simulink model "SecRwLtStLtwdRtwdTrgtPosSelc"  (R2018b)
settings: Solver=FixedStepDiscrete  StartTime=0.0  StopTime=10.0  FixedStep=0.01  RelTol=1e-3
undefined symbols (not defined in the file or in its folder): KeSMSw6sAcsEntrySecRwLtStLtwdRtwdPos_Val, KeSMSw6sAcsEntrySecRwLtStLtwdRtwdPosMax_Val, KeSMSw6sAcsEntrySecRwLtStLtwdRtwdPosMin_Val, KeSMSw6sAcsExtSecRwLtStLtwdRtwdPos_Val, KeSMSw6sAcsExtSecRwLtStLtwdRtwdPosMax_Val, KeSMSw6sAcsExtSecRwLtStLtwdRtwdPosMin_Val, KeSMSw6sFamilyMdSecRwLtStLtwdRtwdPos_Val, KeSMSw6sFamilyMdSecRwLtStLtwdRtwdPosMax_Val, KeSMSw6sFamilyMdSecRwLtStLtwdRtwdPosMin_Val, KeSMSw6sFamilyRMdSecRwLtStLtwdRtwdPos_Val, KeSMSw6sFamilyRMdSecRwLtStLtwdRtwdPosMax_Val, KeSMSw6sFamilyRMdSecRwLtStLtwdRtwdPosMin_Val, KeSMSw6sIntimacyMdSecRwLtStLtwdRtwdPos_Val, KeSMSw6sIntimacyMdSecRwLtStLtwdRtwdPosMax_Val, KeSMSw6sIntimacyMdSecRwLtStLtwdRtwdPosMin_Val, KeSMSw6sIntimacyRMdSecRwLtStLtwdRtwdPos_Val, KeSMSw6sIntimacyRMdSecRwLtStLtwdRtwdPosMax_Val, KeSMSw6sIntimacyRMdSecRwLtStLtwdRtwdPosMin_Val, KeSMSw6sVIPSecRwLtStLtwdRtwdPos_Val, KeSMSw6sVIPSecRwLtStLtwdRtwdPosMax_Val, KeSMSw6sVIPSecRwLtStLtwdRtwdPosMin_Val, KeSMSwAcsEntrySecRwLtStLtwdRtwdPos_Val, KeSMSwAcsEntrySecRwLtStLtwdRtwdPosMax_Val, KeSMSwAcsEntrySecRwLtStLtwdRtwdPosMin_Val, KeSMSwAcsExtSecRwLtStLtwdRtwdPos_Val, KeSMSwAcsExtSecRwLtStLtwdRtwdPosMax_Val, KeSMSwAcsExtSecRwLtStLtwdRtwdPosMin_Val, KeSMSwFamilyMdSecRwLtStLtwdRtwdPos_Val, KeSMSwFamilyMdSecRwLtStLtwdRtwdPosMax_Val, KeSMSwFamilyMdSecRwLtStLtwdRtwdPosMin_Val, KeSMSwFamilyRMdSecRwLtStLtwdRtwdPos_Val, KeSMSwFamilyRMdSecRwLtStLtwdRtwdPosMax_Val, KeSMSwFamilyRMdSecRwLtStLtwdRtwdPosMin_Val, KeSMSwIntimacyMdSecRwLtStLtwdRtwdPos_Val, KeSMSwIntimacyMdSecRwLtStLtwdRtwdPosMax_Val, KeSMSwIntimacyMdSecRwLtStLtwdRtwdPosMin_Val, KeSMSwIntimacyRMdSecRwLtStLtwdRtwdPos_Val, KeSMSwIntimacyRMdSecRwLtStLtwdRtwdPosMax_Val, KeSMSwIntimacyRMdSecRwLtStLtwdRtwdPosMin_Val, KeSMSwVIPSecRwLtStLtwdRtwdPos_Val, KeSMSwVIPSecRwLtStLtwdRtwdPosMax_Val, KeSMSwVIPSecRwLtStLtwdRtwdPosMin_Val
libraries: TrgtPosSelcLib x8
settings Model: Creator=sn2xws  LastModifiedBy=sn2xws
settings DataIOCC: SaveFormat=StructureWithTime
settings OptimizationCC: DefaultParameterBehavior=Inlined  EnhancedBackFolding=on  PassReuseOutputArgsAs=Individual arguments  ZeroExternalMemoryAtStartup=off  ZeroInternalMemoryAtStartup=off  OptimizeBlockOrder=speed  DifferentSizesBufferReuse=on  OptimizationCustomize=off
settings DebuggingCC: ParameterTunabilityLossMsg=error
settings ModelReferenceCC: ModelReferenceNumInstancesAllowed=Single
settings SFSimCC: MATLABDynamicMemAlloc=off
settings RTWCC: SystemTargetFile=autosar.tlc  GenCodeOnly=on  TemplateMakefile=ert_default_tmf  Description=AUTOSAR  GenerateReport=on  IncludeHyperlinkInReport=on  LaunchReport=on  GenerateTraceInfo=on  GenerateTraceReport=on  GenerateTraceReportSl=on  GenerateTraceReportSf=on  GenerateTraceReportEml=on
settings CodeAppCC: ForceParamTrailComments=on  IgnoreCustomStorageClasses=off  OperatorAnnotations=on  SimulinkDataObjDesc=on  SFDataObjDesc=on  InsertBlockDesc=on
settings STFCustomTargetCC: TargetLangStandard=C99 (ISO)  MultiwordLength=256  ParMdlRefBuildCompliant=on  CompOptLevelCompliant=on  IncludeMdlTerminateFcn=off  CombineOutputUpdateFcns=on  SuppressErrorStatus=on  ERTCustomFileBanners=on  SupportNonFinite=off  SupportComplex=off  SupportContinuousTime=off  SupportNonInlinedSFcns=off  RemoveResetFunc=on  MATLABClassNameForMDSCustomization=Simulink.SoftwareTarget.ERTCustomization  AutosarCompliant=on  UseToolchainInfoCompliant=on  LookupTableObjectStructAxisOrder=2,1,3,4,...  LUTObjectStructOrderEvenSpacing=Size,Table,Breakpoints  SystemTargetFile=autosar.tlc
settings ERTTargetCC: TargetLangStandard=C99 (ISO)  ConcurrentExecutionCompliant=off  IncludeMdlTerminateFcn=off  SuppressErrorStatus=on  SupportNonFinite=off  SupportComplex=off  ModelStepFunctionPrototypeControlCompliant=off  CPPClassGenCompliant=off  AutosarCompliant=on  LookupTableObjectStructAxisOrder=2,1,3,4,...  LUTObjectStructOrderEvenSpacing=Size,Table,Breakpoints  InlinedParameterPlacement=NonHierarchical  ERTCustomFileTemplate=example_file_process.tlc  ERTFilePackagingFormat=Compact

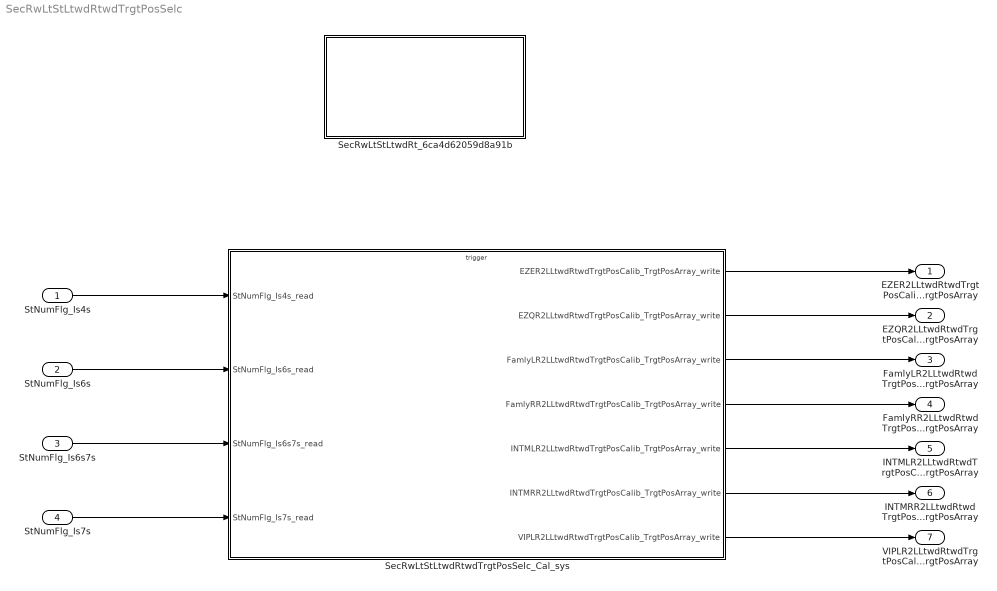
== system SecRwLtStLtwdRtwdTrgtPosSelc ==
  StNumFlg_Is4s : Inport  OutDataTypeStr=boolean  PortDimensions=1
  StNumFlg_Is6s : Inport  Port=2  OutDataTypeStr=boolean  PortDimensions=1
  StNumFlg_Is6s7s : Inport  Port=3  OutDataTypeStr=boolean  PortDimensions=1
  StNumFlg_Is7s : Inport  Port=4  OutDataTypeStr=boolean  PortDimensions=1
  SecRwLtStLtwdRt_6ca4d62059d8a91b : Subsystem
  SecRwLtStLtwdRtwdTrgtPosSelc_Cal_sys : Subsystem
  EZER2LLtwdRtwdTrgtPosCalib_TrgtPosArray : Outport  Description=|  OutDataTypeStr=uint16  PortDimensions=3
      | 0:Pos
      | 1:Max
      | 2:Min
  EZQR2LLtwdRtwdTrgtPosCalib_TrgtPosArray : Outport  Description=|  Port=2  OutDataTypeStr=uint16  PortDimensions=3
      | 0:Pos
      | 1:Max
      | 2:Min
  FamlyLR2LLtwdRtwdTrgtPosCalib_TrgtPosArray : Outport  Description=|  Port=3  OutDataTypeStr=uint16  PortDimensions=3
      | 0:Pos
      | 1:Max
      | 2:Min
  FamlyRR2LLtwdRtwdTrgtPosCalib_TrgtPosArray : Outport  Description=|  Port=4  OutDataTypeStr=uint16  PortDimensions=3
      | 0:Pos
      | 1:Max
      | 2:Min
  INTMLR2LLtwdRtwdTrgtPosCalib_TrgtPosArray : Outport  Description=|  Port=5  OutDataTypeStr=uint16  PortDimensions=3
      | 0:Pos
      | 1:Max
      | 2:Min
  INTMRR2LLtwdRtwdTrgtPosCalib_TrgtPosArray : Outport  Description=|  Port=6  OutDataTypeStr=uint16  PortDimensions=3
      | 0:Pos
      | 1:Max
      | 2:Min
  VIPLR2LLtwdRtwdTrgtPosCalib_TrgtPosArray : Outport  Description=|  Port=7  OutDataTypeStr=uint16  PortDimensions=3
      | 0:Pos
      | 1:Max
      | 2:Min
  wires:
  StNumFlg_Is4s/1 -> SecRwLtStLtwdRtwdTrgtPosSelc_Cal_sys/1(StNumFlg_Is4s_read)
  StNumFlg_Is6s/1 -> SecRwLtStLtwdRtwdTrgtPosSelc_Cal_sys/2(StNumFlg_Is6s_read)
  StNumFlg_Is6s7s/1 -> SecRwLtStLtwdRtwdTrgtPosSelc_Cal_sys/3(StNumFlg_Is6s7s_read)
  StNumFlg_Is7s/1 -> SecRwLtStLtwdRtwdTrgtPosSelc_Cal_sys/4(StNumFlg_Is7s_read)
  SecRwLtStLtwdRtwdTrgtPosSelc_Cal_sys/1(EZER2LLtwdRtwdTrgtPosCalib_TrgtPosArray_write) -> EZER2LLtwdRtwdTrgtPosCalib_TrgtPosArray/1
  SecRwLtStLtwdRtwdTrgtPosSelc_Cal_sys/2(EZQR2LLtwdRtwdTrgtPosCalib_TrgtPosArray_write) -> EZQR2LLtwdRtwdTrgtPosCalib_TrgtPosArray/1
  SecRwLtStLtwdRtwdTrgtPosSelc_Cal_sys/3(FamlyLR2LLtwdRtwdTrgtPosCalib_TrgtPosArray_write) -> FamlyLR2LLtwdRtwdTrgtPosCalib_TrgtPosArray/1
  SecRwLtStLtwdRtwdTrgtPosSelc_Cal_sys/4(FamlyRR2LLtwdRtwdTrgtPosCalib_TrgtPosArray_write) -> FamlyRR2LLtwdRtwdTrgtPosCalib_TrgtPosArray/1
  SecRwLtStLtwdRtwdTrgtPosSelc_Cal_sys/5(INTMLR2LLtwdRtwdTrgtPosCalib_TrgtPosArray_write) -> INTMLR2LLtwdRtwdTrgtPosCalib_TrgtPosArray/1
  SecRwLtStLtwdRtwdTrgtPosSelc_Cal_sys/6(INTMRR2LLtwdRtwdTrgtPosCalib_TrgtPosArray_write) -> INTMRR2LLtwdRtwdTrgtPosCalib_TrgtPosArray/1
  SecRwLtStLtwdRtwdTrgtPosSelc_Cal_sys/7(VIPLR2LLtwdRtwdTrgtPosCalib_TrgtPosArray_write) -> VIPLR2LLtwdRtwdTrgtPosCalib_TrgtPosArray/1

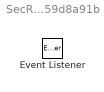
== system SecRwLtStLtwdRtwdTrgtPosSelc/SecRwLtStLtwdRt_6ca4d62059d8a91b ==
  Event Listener : EventListener  EventName=reset

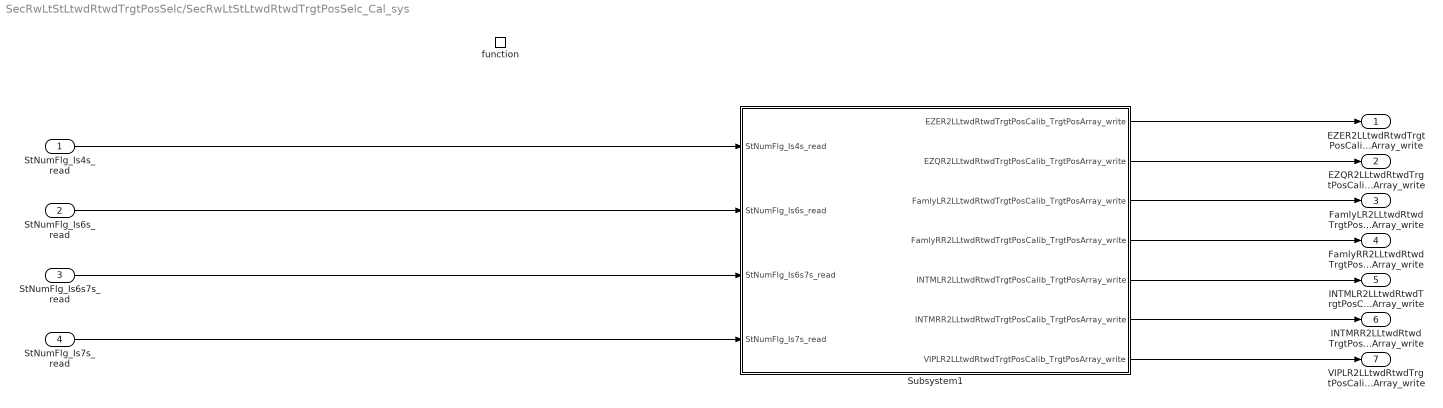
== system SecRwLtStLtwdRtwdTrgtPosSelc/SecRwLtStLtwdRtwdTrgtPosSelc_Cal_sys ==
  StNumFlg_Is4s_read : Inport
  StNumFlg_Is6s_read : Inport  Port=2
  StNumFlg_Is6s7s_read : Inport  Port=3
  StNumFlg_Is7s_read : Inport  Port=4
  function : TriggerPort  TriggerType=function-call  IsSimulinkFunction=on  FunctionName=SecRwLtStLtwdRtwdTrgtPosSelc_Cal  VariantControl=(inherit)
  Subsystem1 : Subsystem
  EZER2LLtwdRtwdTrgtPosCalib_TrgtPosArray_write : Outport
      settings: EnsureOutportIsVirtual=on
  EZQR2LLtwdRtwdTrgtPosCalib_TrgtPosArray_write : Outport  Port=2
      settings: EnsureOutportIsVirtual=on
  FamlyLR2LLtwdRtwdTrgtPosCalib_TrgtPosArray_write : Outport  Port=3
      settings: EnsureOutportIsVirtual=on
  FamlyRR2LLtwdRtwdTrgtPosCalib_TrgtPosArray_write : Outport  Port=4
      settings: EnsureOutportIsVirtual=on
  INTMLR2LLtwdRtwdTrgtPosCalib_TrgtPosArray_write : Outport  Port=5
      settings: EnsureOutportIsVirtual=on
  INTMRR2LLtwdRtwdTrgtPosCalib_TrgtPosArray_write : Outport  Port=6
      settings: EnsureOutportIsVirtual=on
  VIPLR2LLtwdRtwdTrgtPosCalib_TrgtPosArray_write : Outport  Port=7
      settings: EnsureOutportIsVirtual=on
  wires:
  Subsystem1/1(EZER2LLtwdRtwdTrgtPosCalib_TrgtPosArray_write) -> EZER2LLtwdRtwdTrgtPosCalib_TrgtPosArray_write/1
  Subsystem1/2(EZQR2LLtwdRtwdTrgtPosCalib_TrgtPosArray_write) -> EZQR2LLtwdRtwdTrgtPosCalib_TrgtPosArray_write/1
  Subsystem1/3(FamlyLR2LLtwdRtwdTrgtPosCalib_TrgtPosArray_write) -> FamlyLR2LLtwdRtwdTrgtPosCalib_TrgtPosArray_write/1
  Subsystem1/4(FamlyRR2LLtwdRtwdTrgtPosCalib_TrgtPosArray_write) -> FamlyRR2LLtwdRtwdTrgtPosCalib_TrgtPosArray_write/1
  Subsystem1/5(INTMLR2LLtwdRtwdTrgtPosCalib_TrgtPosArray_write) -> INTMLR2LLtwdRtwdTrgtPosCalib_TrgtPosArray_write/1
  Subsystem1/6(INTMRR2LLtwdRtwdTrgtPosCalib_TrgtPosArray_write) -> INTMRR2LLtwdRtwdTrgtPosCalib_TrgtPosArray_write/1
  Subsystem1/7(VIPLR2LLtwdRtwdTrgtPosCalib_TrgtPosArray_write) -> VIPLR2LLtwdRtwdTrgtPosCalib_TrgtPosArray_write/1
  StNumFlg_Is4s_read/1 -> Subsystem1/1(StNumFlg_Is4s_read)
  StNumFlg_Is6s_read/1 -> Subsystem1/2(StNumFlg_Is6s_read)
  StNumFlg_Is6s7s_read/1 -> Subsystem1/3(StNumFlg_Is6s7s_read)
  StNumFlg_Is7s_read/1 -> Subsystem1/4(StNumFlg_Is7s_read)

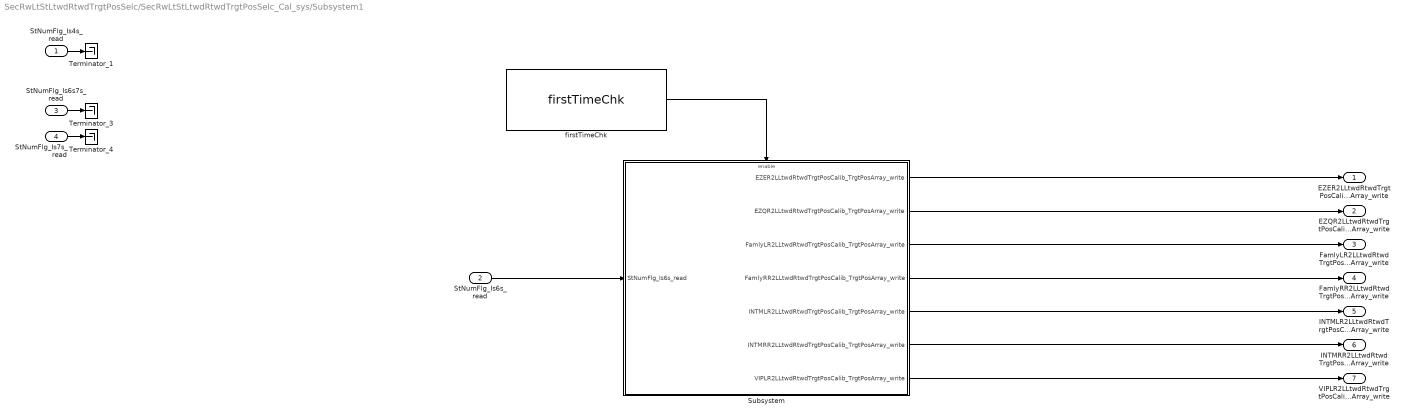
== system SecRwLtStLtwdRtwdTrgtPosSelc/SecRwLtStLtwdRtwdTrgtPosSelc_Cal_sys/Subsystem1 ==
  StNumFlg_Is4s_read : Inport
  StNumFlg_Is6s_read : Inport  Port=2
  StNumFlg_Is6s7s_read : Inport  Port=3
  StNumFlg_Is7s_read : Inport  Port=4
  Subsystem : Subsystem
  Terminator_1 : Terminator
  Terminator_3 : Terminator
  Terminator_4 : Terminator
  firstTimeChk : TrgtPosSelcLib/firstTimeChk  SystemSampleTime=-1
  EZER2LLtwdRtwdTrgtPosCalib_TrgtPosArray_write : Outport
      settings: EnsureOutportIsVirtual=on
  EZQR2LLtwdRtwdTrgtPosCalib_TrgtPosArray_write : Outport  Port=2
      settings: EnsureOutportIsVirtual=on
  FamlyLR2LLtwdRtwdTrgtPosCalib_TrgtPosArray_write : Outport  Port=3
      settings: EnsureOutportIsVirtual=on
  FamlyRR2LLtwdRtwdTrgtPosCalib_TrgtPosArray_write : Outport  Port=4
      settings: EnsureOutportIsVirtual=on
  INTMLR2LLtwdRtwdTrgtPosCalib_TrgtPosArray_write : Outport  Port=5
      settings: EnsureOutportIsVirtual=on
  INTMRR2LLtwdRtwdTrgtPosCalib_TrgtPosArray_write : Outport  Port=6
      settings: EnsureOutportIsVirtual=on
  VIPLR2LLtwdRtwdTrgtPosCalib_TrgtPosArray_write : Outport  Port=7
      settings: EnsureOutportIsVirtual=on
  wires:
  StNumFlg_Is4s_read/1 -> Terminator_1/1
  StNumFlg_Is6s7s_read/1 -> Terminator_3/1
  Subsystem/6(INTMRR2LLtwdRtwdTrgtPosCalib_TrgtPosArray_write) -> INTMRR2LLtwdRtwdTrgtPosCalib_TrgtPosArray_write/1
  Subsystem/3(FamlyLR2LLtwdRtwdTrgtPosCalib_TrgtPosArray_write) -> FamlyLR2LLtwdRtwdTrgtPosCalib_TrgtPosArray_write/1
  Subsystem/1(EZER2LLtwdRtwdTrgtPosCalib_TrgtPosArray_write) -> EZER2LLtwdRtwdTrgtPosCalib_TrgtPosArray_write/1
  Subsystem/2(EZQR2LLtwdRtwdTrgtPosCalib_TrgtPosArray_write) -> EZQR2LLtwdRtwdTrgtPosCalib_TrgtPosArray_write/1
  Subsystem/5(INTMLR2LLtwdRtwdTrgtPosCalib_TrgtPosArray_write) -> INTMLR2LLtwdRtwdTrgtPosCalib_TrgtPosArray_write/1
  Subsystem/4(FamlyRR2LLtwdRtwdTrgtPosCalib_TrgtPosArray_write) -> FamlyRR2LLtwdRtwdTrgtPosCalib_TrgtPosArray_write/1
  Subsystem/7(VIPLR2LLtwdRtwdTrgtPosCalib_TrgtPosArray_write) -> VIPLR2LLtwdRtwdTrgtPosCalib_TrgtPosArray_write/1
  StNumFlg_Is7s_read/1 -> Terminator_4/1
  StNumFlg_Is6s_read/1 -> Subsystem/1(StNumFlg_Is6s_read)
  firstTimeChk/1 -> Subsystem/Enable

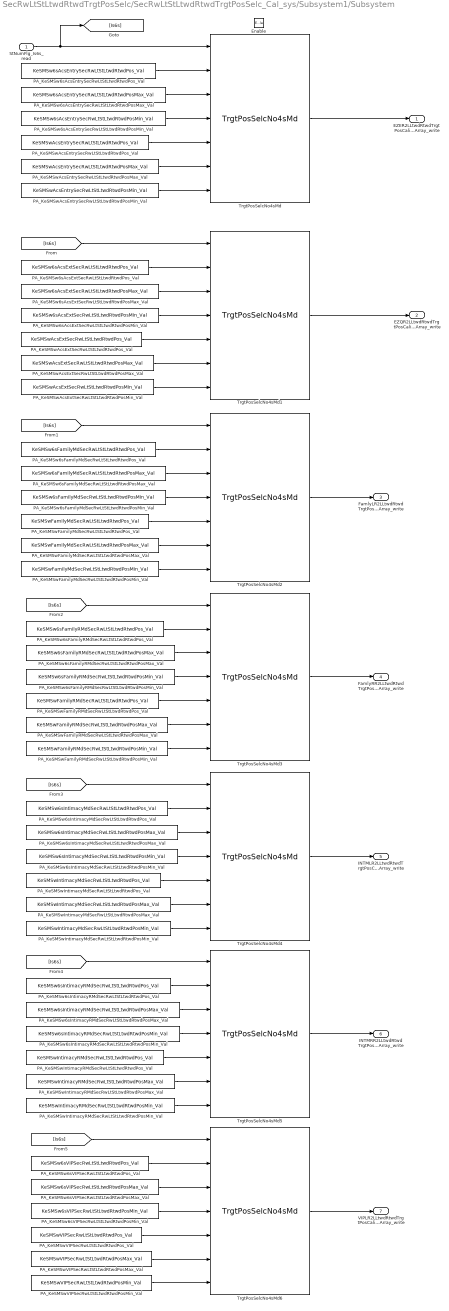
== system SecRwLtStLtwdRtwdTrgtPosSelc/SecRwLtStLtwdRtwdTrgtPosSelc_Cal_sys/Subsystem1/Subsystem ==
  StNumFlg_Is6s_read : Inport
  Enable : EnablePort
  PA_KeSMSw6sAcsEntrySecRwLtStLtwdRtwdPosMax_Val : Constant  Value=KeSMSw6sAcsEntrySecRwLtStLtwdRtwdPosMax_Val
  PA_KeSMSw6sAcsEntrySecRwLtStLtwdRtwdPosMin_Val : Constant  Value=KeSMSw6sAcsEntrySecRwLtStLtwdRtwdPosMin_Val
  PA_KeSMSw6sAcsEntrySecRwLtStLtwdRtwdPos_Val : Constant  Value=KeSMSw6sAcsEntrySecRwLtStLtwdRtwdPos_Val
  PA_KeSMSw6sAcsExtSecRwLtStLtwdRtwdPosMax_Val : Constant  Value=KeSMSw6sAcsExtSecRwLtStLtwdRtwdPosMax_Val
  PA_KeSMSw6sAcsExtSecRwLtStLtwdRtwdPosMin_Val : Constant  Value=KeSMSw6sAcsExtSecRwLtStLtwdRtwdPosMin_Val
  PA_KeSMSw6sAcsExtSecRwLtStLtwdRtwdPos_Val : Constant  Value=KeSMSw6sAcsExtSecRwLtStLtwdRtwdPos_Val
  PA_KeSMSw6sFamilyMdSecRwLtStLtwdRtwdPosMax_Val : Constant  Value=KeSMSw6sFamilyMdSecRwLtStLtwdRtwdPosMax_Val
  PA_KeSMSw6sFamilyMdSecRwLtStLtwdRtwdPosMin_Val : Constant  Value=KeSMSw6sFamilyMdSecRwLtStLtwdRtwdPosMin_Val
  PA_KeSMSw6sFamilyMdSecRwLtStLtwdRtwdPos_Val : Constant  Value=KeSMSw6sFamilyMdSecRwLtStLtwdRtwdPos_Val
  PA_KeSMSw6sFamilyRMdSecRwLtStLtwdRtwdPosMax_Val : Constant  Value=KeSMSw6sFamilyRMdSecRwLtStLtwdRtwdPosMax_Val
  PA_KeSMSw6sFamilyRMdSecRwLtStLtwdRtwdPosMin_Val : Constant  Value=KeSMSw6sFamilyRMdSecRwLtStLtwdRtwdPosMin_Val
  PA_KeSMSw6sFamilyRMdSecRwLtStLtwdRtwdPos_Val : Constant  Value=KeSMSw6sFamilyRMdSecRwLtStLtwdRtwdPos_Val
  PA_KeSMSw6sIntimacyMdSecRwLtStLtwdRtwdPosMax_Val : Constant  Value=KeSMSw6sIntimacyMdSecRwLtStLtwdRtwdPosMax_Val
  PA_KeSMSw6sIntimacyMdSecRwLtStLtwdRtwdPosMin_Val : Constant  Value=KeSMSw6sIntimacyMdSecRwLtStLtwdRtwdPosMin_Val
  PA_KeSMSw6sIntimacyMdSecRwLtStLtwdRtwdPos_Val : Constant  Value=KeSMSw6sIntimacyMdSecRwLtStLtwdRtwdPos_Val
  PA_KeSMSw6sIntimacyRMdSecRwLtStLtwdRtwdPosMax_Val : Constant  Value=KeSMSw6sIntimacyRMdSecRwLtStLtwdRtwdPosMax_Val
  PA_KeSMSw6sIntimacyRMdSecRwLtStLtwdRtwdPosMin_Val : Constant  Value=KeSMSw6sIntimacyRMdSecRwLtStLtwdRtwdPosMin_Val
  PA_KeSMSw6sIntimacyRMdSecRwLtStLtwdRtwdPos_Val : Constant  Value=KeSMSw6sIntimacyRMdSecRwLtStLtwdRtwdPos_Val
  PA_KeSMSw6sVIPSecRwLtStLtwdRtwdPosMax_Val : Constant  Value=KeSMSw6sVIPSecRwLtStLtwdRtwdPosMax_Val
  PA_KeSMSw6sVIPSecRwLtStLtwdRtwdPosMin_Val : Constant  Value=KeSMSw6sVIPSecRwLtStLtwdRtwdPosMin_Val
  PA_KeSMSw6sVIPSecRwLtStLtwdRtwdPos_Val : Constant  Value=KeSMSw6sVIPSecRwLtStLtwdRtwdPos_Val
  PA_KeSMSwAcsEntrySecRwLtStLtwdRtwdPosMax_Val : Constant  Value=KeSMSwAcsEntrySecRwLtStLtwdRtwdPosMax_Val
  PA_KeSMSwAcsEntrySecRwLtStLtwdRtwdPosMin_Val : Constant  Value=KeSMSwAcsEntrySecRwLtStLtwdRtwdPosMin_Val
  PA_KeSMSwAcsEntrySecRwLtStLtwdRtwdPos_Val : Constant  Value=KeSMSwAcsEntrySecRwLtStLtwdRtwdPos_Val
  PA_KeSMSwAcsExtSecRwLtStLtwdRtwdPosMax_Val : Constant  Value=KeSMSwAcsExtSecRwLtStLtwdRtwdPosMax_Val
  PA_KeSMSwAcsExtSecRwLtStLtwdRtwdPosMin_Val : Constant  Value=KeSMSwAcsExtSecRwLtStLtwdRtwdPosMin_Val
  PA_KeSMSwAcsExtSecRwLtStLtwdRtwdPos_Val : Constant  Value=KeSMSwAcsExtSecRwLtStLtwdRtwdPos_Val
  PA_KeSMSwFamilyMdSecRwLtStLtwdRtwdPosMax_Val : Constant  Value=KeSMSwFamilyMdSecRwLtStLtwdRtwdPosMax_Val
  PA_KeSMSwFamilyMdSecRwLtStLtwdRtwdPosMin_Val : Constant  Value=KeSMSwFamilyMdSecRwLtStLtwdRtwdPosMin_Val
  PA_KeSMSwFamilyMdSecRwLtStLtwdRtwdPos_Val : Constant  Value=KeSMSwFamilyMdSecRwLtStLtwdRtwdPos_Val
  PA_KeSMSwFamilyRMdSecRwLtStLtwdRtwdPosMax_Val : Constant  Value=KeSMSwFamilyRMdSecRwLtStLtwdRtwdPosMax_Val
  PA_KeSMSwFamilyRMdSecRwLtStLtwdRtwdPosMin_Val : Constant  Value=KeSMSwFamilyRMdSecRwLtStLtwdRtwdPosMin_Val
  PA_KeSMSwFamilyRMdSecRwLtStLtwdRtwdPos_Val : Constant  Value=KeSMSwFamilyRMdSecRwLtStLtwdRtwdPos_Val
  PA_KeSMSwIntimacyMdSecRwLtStLtwdRtwdPosMax_Val : Constant  Value=KeSMSwIntimacyMdSecRwLtStLtwdRtwdPosMax_Val
  PA_KeSMSwIntimacyMdSecRwLtStLtwdRtwdPosMin_Val : Constant  Value=KeSMSwIntimacyMdSecRwLtStLtwdRtwdPosMin_Val
  PA_KeSMSwIntimacyMdSecRwLtStLtwdRtwdPos_Val : Constant  Value=KeSMSwIntimacyMdSecRwLtStLtwdRtwdPos_Val
  PA_KeSMSwIntimacyRMdSecRwLtStLtwdRtwdPosMax_Val : Constant  Value=KeSMSwIntimacyRMdSecRwLtStLtwdRtwdPosMax_Val
  PA_KeSMSwIntimacyRMdSecRwLtStLtwdRtwdPosMin_Val : Constant  Value=KeSMSwIntimacyRMdSecRwLtStLtwdRtwdPosMin_Val
  PA_KeSMSwIntimacyRMdSecRwLtStLtwdRtwdPos_Val : Constant  Value=KeSMSwIntimacyRMdSecRwLtStLtwdRtwdPos_Val
  PA_KeSMSwVIPSecRwLtStLtwdRtwdPosMax_Val : Constant  Value=KeSMSwVIPSecRwLtStLtwdRtwdPosMax_Val
  PA_KeSMSwVIPSecRwLtStLtwdRtwdPosMin_Val : Constant  Value=KeSMSwVIPSecRwLtStLtwdRtwdPosMin_Val
  PA_KeSMSwVIPSecRwLtStLtwdRtwdPos_Val : Constant  Value=KeSMSwVIPSecRwLtStLtwdRtwdPos_Val
  TrgtPosSelcNo4sMd{,1..6} (7 alike) : TrgtPosSelcLib/TrgtPosSelcNo4sMd  SystemSampleTime=-1
  EZER2LLtwdRtwdTrgtPosCalib_TrgtPosArray_write : Outport
      settings: EnsureOutportIsVirtual=on
  EZQR2LLtwdRtwdTrgtPosCalib_TrgtPosArray_write : Outport  Port=2
      settings: EnsureOutportIsVirtual=on
  FamlyLR2LLtwdRtwdTrgtPosCalib_TrgtPosArray_write : Outport  Port=3
      settings: EnsureOutportIsVirtual=on
  FamlyRR2LLtwdRtwdTrgtPosCalib_TrgtPosArray_write : Outport  Port=4
      settings: EnsureOutportIsVirtual=on
  INTMLR2LLtwdRtwdTrgtPosCalib_TrgtPosArray_write : Outport  Port=5
      settings: EnsureOutportIsVirtual=on
  INTMRR2LLtwdRtwdTrgtPosCalib_TrgtPosArray_write : Outport  Port=6
      settings: EnsureOutportIsVirtual=on
  VIPLR2LLtwdRtwdTrgtPosCalib_TrgtPosArray_write : Outport  Port=7
      settings: EnsureOutportIsVirtual=on
  wires:
  PA_KeSMSw6sAcsEntrySecRwLtStLtwdRtwdPosMin_Val/1 -> TrgtPosSelcNo4sMd/4
  [Is6s] -> TrgtPosSelcNo4sMd5/1
  PA_KeSMSw6sAcsEntrySecRwLtStLtwdRtwdPosMax_Val/1 -> TrgtPosSelcNo4sMd/3
  TrgtPosSelcNo4sMd5/1 -> INTMRR2LLtwdRtwdTrgtPosCalib_TrgtPosArray_write/1
  TrgtPosSelcNo4sMd/1 -> EZER2LLtwdRtwdTrgtPosCalib_TrgtPosArray_write/1
  PA_KeSMSw6sIntimacyMdSecRwLtStLtwdRtwdPosMin_Val/1 -> TrgtPosSelcNo4sMd4/4
  PA_KeSMSwFamilyMdSecRwLtStLtwdRtwdPosMin_Val/1 -> TrgtPosSelcNo4sMd2/7
  PA_KeSMSwIntimacyRMdSecRwLtStLtwdRtwdPosMin_Val/1 -> TrgtPosSelcNo4sMd5/7
  PA_KeSMSw6sFamilyMdSecRwLtStLtwdRtwdPos_Val/1 -> TrgtPosSelcNo4sMd2/2
  PA_KeSMSw6sFamilyRMdSecRwLtStLtwdRtwdPosMax_Val/1 -> TrgtPosSelcNo4sMd3/3
  PA_KeSMSw6sAcsEntrySecRwLtStLtwdRtwdPos_Val/1 -> TrgtPosSelcNo4sMd/2
  TrgtPosSelcNo4sMd6/1 -> VIPLR2LLtwdRtwdTrgtPosCalib_TrgtPosArray_write/1
  PA_KeSMSwFamilyRMdSecRwLtStLtwdRtwdPosMin_Val/1 -> TrgtPosSelcNo4sMd3/7
  TrgtPosSelcNo4sMd1/1 -> EZQR2LLtwdRtwdTrgtPosCalib_TrgtPosArray_write/1
  PA_KeSMSwFamilyRMdSecRwLtStLtwdRtwdPosMax_Val/1 -> TrgtPosSelcNo4sMd3/6
  PA_KeSMSwIntimacyRMdSecRwLtStLtwdRtwdPos_Val/1 -> TrgtPosSelcNo4sMd5/5
  PA_KeSMSw6sFamilyRMdSecRwLtStLtwdRtwdPosMin_Val/1 -> TrgtPosSelcNo4sMd3/4
  TrgtPosSelcNo4sMd3/1 -> FamlyRR2LLtwdRtwdTrgtPosCalib_TrgtPosArray_write/1
  TrgtPosSelcNo4sMd4/1 -> INTMLR2LLtwdRtwdTrgtPosCalib_TrgtPosArray_write/1
  PA_KeSMSwFamilyMdSecRwLtStLtwdRtwdPosMax_Val/1 -> TrgtPosSelcNo4sMd2/6
  PA_KeSMSwVIPSecRwLtStLtwdRtwdPos_Val/1 -> TrgtPosSelcNo4sMd6/5
  PA_KeSMSwFamilyMdSecRwLtStLtwdRtwdPos_Val/1 -> TrgtPosSelcNo4sMd2/5
  PA_KeSMSwIntimacyRMdSecRwLtStLtwdRtwdPosMax_Val/1 -> TrgtPosSelcNo4sMd5/6
  [Is6s] -> TrgtPosSelcNo4sMd4/1
  PA_KeSMSwVIPSecRwLtStLtwdRtwdPosMin_Val/1 -> TrgtPosSelcNo4sMd6/7
  PA_KeSMSw6sFamilyMdSecRwLtStLtwdRtwdPosMin_Val/1 -> TrgtPosSelcNo4sMd2/4
  PA_KeSMSw6sVIPSecRwLtStLtwdRtwdPos_Val/1 -> TrgtPosSelcNo4sMd6/2
  PA_KeSMSw6sVIPSecRwLtStLtwdRtwdPosMin_Val/1 -> TrgtPosSelcNo4sMd6/4
  PA_KeSMSw6sIntimacyMdSecRwLtStLtwdRtwdPosMax_Val/1 -> TrgtPosSelcNo4sMd4/3
  [Is6s] -> TrgtPosSelcNo4sMd2/1
  PA_KeSMSw6sAcsExtSecRwLtStLtwdRtwdPos_Val/1 -> TrgtPosSelcNo4sMd1/2
  PA_KeSMSw6sVIPSecRwLtStLtwdRtwdPosMax_Val/1 -> TrgtPosSelcNo4sMd6/3
  PA_KeSMSwAcsExtSecRwLtStLtwdRtwdPos_Val/1 -> TrgtPosSelcNo4sMd1/5
  PA_KeSMSw6sFamilyMdSecRwLtStLtwdRtwdPosMax_Val/1 -> TrgtPosSelcNo4sMd2/3
  PA_KeSMSwFamilyRMdSecRwLtStLtwdRtwdPos_Val/1 -> TrgtPosSelcNo4sMd3/5
  [Is6s] -> TrgtPosSelcNo4sMd1/1
  PA_KeSMSwAcsEntrySecRwLtStLtwdRtwdPos_Val/1 -> TrgtPosSelcNo4sMd/5
  [Is6s] -> TrgtPosSelcNo4sMd6/1
  StNumFlg_Is6s_read/1 -> [Is6s], TrgtPosSelcNo4sMd/1
  PA_KeSMSw6sIntimacyRMdSecRwLtStLtwdRtwdPosMax_Val/1 -> TrgtPosSelcNo4sMd5/3
  PA_KeSMSw6sIntimacyMdSecRwLtStLtwdRtwdPos_Val/1 -> TrgtPosSelcNo4sMd4/2
  PA_KeSMSw6sIntimacyRMdSecRwLtStLtwdRtwdPos_Val/1 -> TrgtPosSelcNo4sMd5/2
  PA_KeSMSw6sIntimacyRMdSecRwLtStLtwdRtwdPosMin_Val/1 -> TrgtPosSelcNo4sMd5/4
  PA_KeSMSw6sAcsExtSecRwLtStLtwdRtwdPosMax_Val/1 -> TrgtPosSelcNo4sMd1/3
  PA_KeSMSw6sFamilyRMdSecRwLtStLtwdRtwdPos_Val/1 -> TrgtPosSelcNo4sMd3/2
  PA_KeSMSwVIPSecRwLtStLtwdRtwdPosMax_Val/1 -> TrgtPosSelcNo4sMd6/6
  [Is6s] -> TrgtPosSelcNo4sMd3/1
  PA_KeSMSwAcsExtSecRwLtStLtwdRtwdPosMax_Val/1 -> TrgtPosSelcNo4sMd1/6
  PA_KeSMSwAcsExtSecRwLtStLtwdRtwdPosMin_Val/1 -> TrgtPosSelcNo4sMd1/7
  PA_KeSMSwAcsEntrySecRwLtStLtwdRtwdPosMax_Val/1 -> TrgtPosSelcNo4sMd/6
  PA_KeSMSwAcsEntrySecRwLtStLtwdRtwdPosMin_Val/1 -> TrgtPosSelcNo4sMd/7
  PA_KeSMSw6sAcsExtSecRwLtStLtwdRtwdPosMin_Val/1 -> TrgtPosSelcNo4sMd1/4
  PA_KeSMSwIntimacyMdSecRwLtStLtwdRtwdPosMin_Val/1 -> TrgtPosSelcNo4sMd4/7
  PA_KeSMSwIntimacyMdSecRwLtStLtwdRtwdPosMax_Val/1 -> TrgtPosSelcNo4sMd4/6
  PA_KeSMSwIntimacyMdSecRwLtStLtwdRtwdPos_Val/1 -> TrgtPosSelcNo4sMd4/5
  TrgtPosSelcNo4sMd2/1 -> FamlyLR2LLtwdRtwdTrgtPosCalib_TrgtPosArray_write/1
